simulink model "sim_es2"  (R2022a)
settings: Solver=VariableStepAuto  StartTime=0.0  StopTime=10.0  RelTol=1e-3
values from neighbouring files (symbols this model uses):
  C = minreal((1/Gzas)*(Gcl/(1-Gcl)))    [parte2.m]
  Gzas = tf(num,den,Tc)    [parte2.m]
  Tc = 0.1    [parte2.m]
settings Model: Creator=Stefano  LastModifiedBy=Stefano

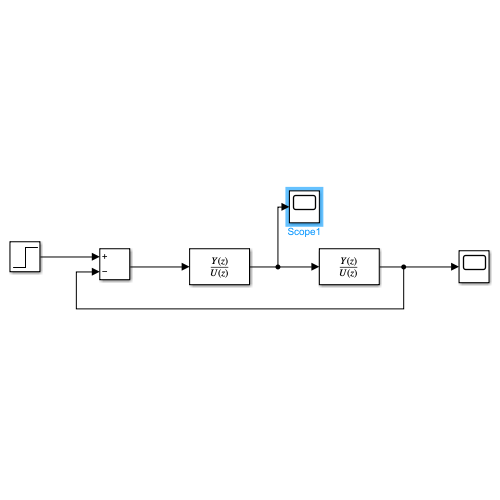
[thumbnail: Simulink's stored preview of the top-level diagram]
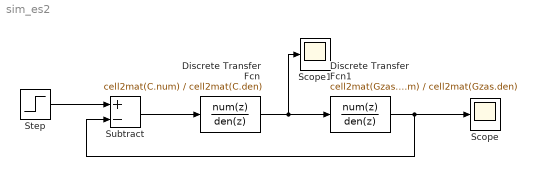
== system sim_es2 ==
  Discrete Transfer Fcn : DiscreteTransferFcn  Numerator=cell2mat(C.num)  Denominator=cell2mat(C.den)  SampleTime=Tc
  Discrete Transfer Fcn1 : DiscreteTransferFcn  Numerator=cell2mat(Gzas.num)  Denominator=cell2mat(Gzas.den)  SampleTime=Tc
  Scope : Scope
  Scope1 : Scope
  Step : Step  SampleTime=0
  Subtract : Sum  Inputs=+-
  wires:
  Discrete Transfer Fcn/1 -> Scope1/1, Discrete Transfer Fcn1/1
  Subtract/1 -> Discrete Transfer Fcn/1
  Step/1 -> Subtract/1
  Discrete Transfer Fcn1/1 -> Scope/1, Subtract/2
